simulink model "control_lqr_integral"  (R2025b)
settings: Solver=ode23t  StartTime=0.0  StopTime=10.0  MaxStep=1e-3  RelTol=1e-3  AbsTol=1e-3
undefined symbols (not defined in the file): K_int, Kf_int, p0
libraries: simulink_extras x2
settings Model: Creator=upattacini  LastModifiedBy=upattacini
settings DataIOCC: SaveOutput=off  DSMLogging=off  SaveTime=off
settings ModelReferenceCC: UpdateModelReferenceTargets=Force

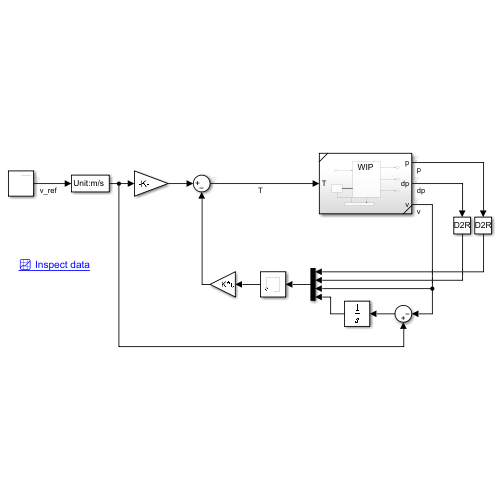
[thumbnail: Simulink's stored preview of the top-level diagram]
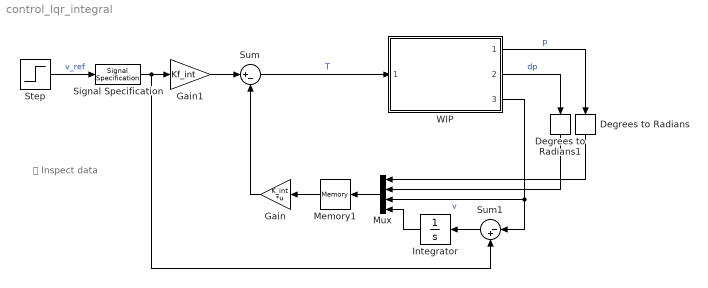
== system control_lqr_integral ==
  note: 📈 Inspect data
  Degrees to Radians : simulink_extras/Transformations/Degrees to Radians
  Degrees to Radians1 : simulink_extras/Transformations/Degrees to Radians
  Gain : Gain  Gain=K_int  Multiplication=Matrix(K*u)
  Gain1 : Gain  Gain=Kf_int
  Integrator : Integrator
  Memory1 : Memory  InitialCondition=[p0*pi/180 0 0 0]  InheritSampleTime=on  LinearizeMemory=on  LinearizeAsDelay=on
  Mux : Mux
  Signal Specification : SignalSpecification  Unit=m/s
  Step : Step  SampleTime=0
  Sum : Sum  Inputs=|+-
  Sum1 : Sum  Inputs=|-+
  WIP : Subsystem  ReferencedSubsystem=WIP
  wires:
  Integrator/1 -> Mux/4
  WIP/3 -> Mux/3, Sum1/1  "v"
  Degrees to Radians/1 -> Mux/1
  Sum1/1 -> Integrator/1
  WIP/2 -> Degrees to Radians1/1  "dp"
  Sum/1 -> WIP/1  "T"
  Signal Specification/1 -> Sum1/2, Gain1/1
  Gain1/1 -> Sum/1
  WIP/1 -> Degrees to Radians/1  "p"
  Memory1/1 -> Gain/1
  Degrees to Radians1/1 -> Mux/2
  Gain/1 -> Sum/2
  Mux/1 -> Memory1/1
  Step/1 -> Signal Specification/1  "v_ref"
